simulink model "simple_puma560controller"  (R2020a)
settings: Solver=VariableStepAuto  StartTime=0.0  StopTime=10.0  RelTol=1e-3
libraries: roblocks x3
settings Model: Creator=yrza  LastModifiedBy=yrza

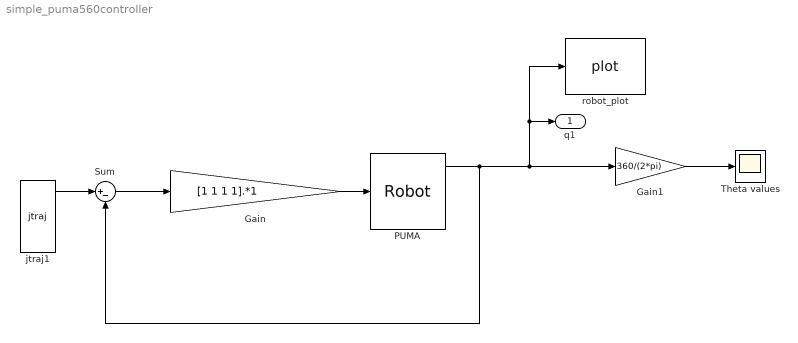
== system simple_puma560controller ==
  Gain : Gain  Gain=[1 1 1 1].*1
  Gain1 : Gain  Gain=360/(2*pi)
  PUMA : roblocks/Arm/Robot  robot=p560  q0=[0 0 0 0 0 0]
  Sum : Sum  Inputs=|+-
  Theta values : Scope
  jtraj1 : roblocks/Toolbox/jtraj  q0=[0 0 0 0 0 0]  qf=[0 pi/2 0 0 0 0]  tmax=10  ts=0.02
  robot_plot : roblocks/Arm/plot  robot=p560  fps=5  holdplot=on
  q1 : Outport
  wires:
  PUMA/1 -> robot_plot/1, q1/1, Gain1/1, Sum/2
  Gain/1 -> PUMA/1
  Gain1/1 -> Theta values/1
  Sum/1 -> Gain/1
  jtraj1/1 -> Sum/1
